simulink model "比例导引"  (R2023b)
settings: Solver=ode4  StartTime=0.0  StopTime=20  FixedStep=0.00005  RelTol=1e-3
settings Model: Creator=PC  LastModifiedBy=PC
settings DataIOCC: ReturnWorkspaceOutputs=off

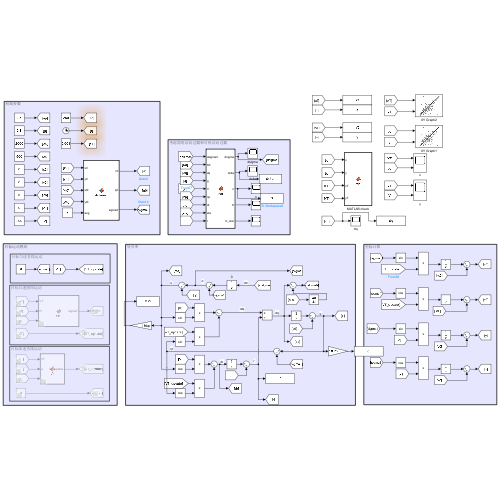
[thumbnail: Simulink's stored preview of the top-level diagram]
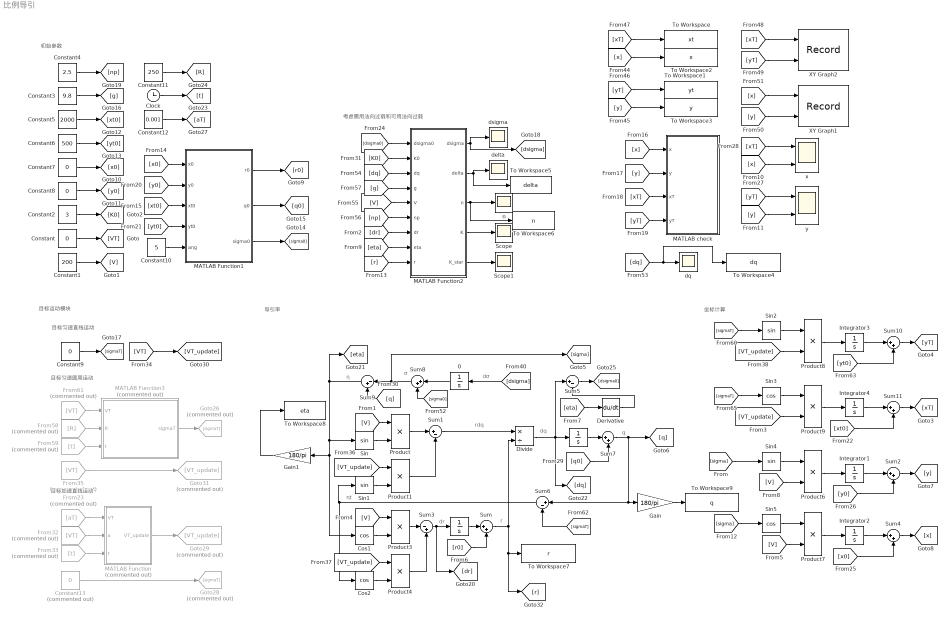
== system 比例导引 ==
  note: 目标加速直线运动
  note: 目标匀速圆周运动
  note: 目标匀速直线运动
  note: 目标运动模块
  note: 初始参数
  note: 导引率
  note: 坐标计算
  note: 考虑需用法向过载和可用法向过载
  note: rdq
  note: σ
  note: q
  note: dσ
  note: dq
  note: r
  note: dr
  note: η
  note: ηt
  " " : Integrator
  "  " : Integrator
  0 : Integrator
  Clock : Clock
  Constant{,7..9} (4 alike) : Constant  Value=0
  Constant1 : Constant  Value=200
  Constant10 : Constant  Value=5
  Constant11 : Constant  Value=250
  Constant12 : Constant  Value=0.001
  Constant13 : Constant  Commented=on  Value=0
  Constant2 : Constant  Value=3
  Constant3 : Constant  Value=9.8
  Constant4 : Constant  Value=2.5
  Constant5 : Constant  Value=2000
  Constant6 : Constant  Value=500
  Cos1 : Trigonometry  Operator=cos
  Cos2 : Trigonometry  Operator=cos
  Derivative : Derivative
  Divide : Product  Inputs=*/
  From23 : From  Commented=on  GotoTag=aT
  From32 : From  Commented=on  GotoTag=VT
  From33 : From  Commented=on  GotoTag=t
  From35 : From  Commented=on  GotoTag=VT
  From58 : From  Commented=on  GotoTag=R
  From59 : From  Commented=on  GotoTag=t
  From61 : From  Commented=on  GotoTag=VT
  Gain : Gain  Gain=180/pi
  Gain1 : Gain  Gain=180/pi
  Goto26 : Goto  Commented=on  GotoTag=sigmaT
  Goto28 : Goto  Commented=on  GotoTag=sigmaT
  Goto29 : Goto  Commented=on  GotoTag=VT_update
  Goto31 : Goto  Commented=on  GotoTag=VT_update
  Integrator{1..4} (4 alike) : Integrator
  MATLAB Function : MATLAB Function  Commented=on  TreatAsAtomicUnit=on
  MATLAB Function1 : MATLAB Function  TreatAsAtomicUnit=on
  MATLAB Function2 : MATLAB Function  TreatAsAtomicUnit=on
  MATLAB Function3 : MATLAB Function  Commented=on  TreatAsAtomicUnit=on
  MATLAB check : MATLAB Function  TreatAsAtomicUnit=on
  Product{,1,3..4,6..9} (8 alike) : Product
  Scope : Scope
  Scope1 : Scope
  Sin{,1..2,4} (4 alike) : Trigonometry
  Sin3 : Trigonometry  Operator=cos
  Sin5 : Trigonometry  Operator=cos
  Sum{,2,4,7..8,10..11} (7 alike) : Sum  Inputs=|++
  Sum1 : Sum  Inputs=|+-
  Sum3 : Sum  Inputs=|-+
  Sum5 : Sum  Inputs=|+-
  Sum6 : Sum  Inputs=|+-
  Sum9 : Sum  Inputs=|-+
  To Workspace : ToWorkspace  VariableName=xt  SaveFormat=Timeseries  SampleTime=-1
  To Workspace1 : ToWorkspace  VariableName=yt  SaveFormat=Timeseries  SampleTime=-1
  To Workspace2 : ToWorkspace  VariableName=x  SaveFormat=Timeseries  SampleTime=-1
  To Workspace3 : ToWorkspace  VariableName=y  SaveFormat=Timeseries  SampleTime=-1
  To Workspace4 : ToWorkspace  VariableName=dq  SaveFormat=Timeseries  SampleTime=-1
  To Workspace5 : ToWorkspace  VariableName=delta  SaveFormat=Timeseries  SampleTime=-1
  To Workspace6 : ToWorkspace  VariableName=n  SaveFormat=Timeseries  SampleTime=-1
  To Workspace7 : ToWorkspace  VariableName=r  SaveFormat=Timeseries  SampleTime=-1
  To Workspace8 : ToWorkspace  VariableName=eta  SaveFormat=Timeseries  SampleTime=-1
  To Workspace9 : ToWorkspace  VariableName=q  SaveFormat=Timeseries  SampleTime=-1
  XY Graph1 : Record  FileSettingsInternal="{\"entries\":[{\"content\":{\"excelSettings\":{\"content\":{},\"type\":\"Streamout.ExcelSettings\"}},\"type\":\"Streamout.FileSettingStorage\",\"uuid\":\"\"}],\"packageUris\":[\"http:\\/\\/schema.mathworks.com\\/mf0\\/streamout_blocks\\/R2020a\"],\"version\":\"1.0\"}"  Layout=[1 1]  SignalsInternal="{\"entries\":[{\"content\":{\"signals\":[{\"content\":{\"blockPath\":[],\"dimensions\":[1],\"domain\":\"\",\"lineColor\":\"#edb120\",\"plots\":[1],\"port\":1,\"sid\":[\"\"],\"signalID\":16369,\"signalName\":\"From51\"},\"type\":\"RecordBlkView.Signal\",\"uuid\":\"\"},{\"content\":{\"blockPath\":[],\"dimensions\":[1],\"domain\":\"\",\"lineColor\":\"#7e2f8e\",\"plots\":[1],\"port\":2,\"sid\":[\"\"],\"signalID\":16373,\"signalName\":\"From50\"},\"type\":\"RecordBlkView.Signal\",\"uuid\":\"\"}]},\"type\":\"RecordBlkView.InputSignals\",\"uuid\":\"\"}],\"packageUris\":[\"http:\\/\\/schema.mathworks.com\\/mf0\\/streamout_blocks\\/R2020a\"],\"version\":\"1.0\"}"  VisualizationBindings="{\"xyplotplugin\":{\"info\":[{\"series\":[{\"bindingParametersList\":[{\"parameter\":\"X-Axis\",\"signalID\":16369,\"signalName\":\"From51\"},{\"parameter\":\"Y-Axis\",\"signalID\":16373,\"signalName\":\"From50\"}],\"seriesID\":6684}],\"subplotID\":1}]}}"  CompatibilityTag=XY
  XY Graph2 : Record  FileSettingsInternal="{\"entries\":[{\"content\":{\"excelSettings\":{\"content\":{},\"type\":\"Streamout.ExcelSettings\"}},\"type\":\"Streamout.FileSettingStorage\",\"uuid\":\"\"}],\"packageUris\":[\"http:\\/\\/schema.mathworks.com\\/mf0\\/streamout_blocks\\/R2020a\"],\"version\":\"1.0\"}"  Layout=[1 1]  SignalsInternal="{\"entries\":[{\"content\":{\"signals\":[{\"content\":{\"blockPath\":[],\"dimensions\":[1],\"domain\":\"\",\"lineColor\":\"#edb120\",\"plots\":[1],\"port\":1,\"sid\":[\"\"],\"signalID\":16377,\"signalName\":\"From48\"},\"type\":\"RecordBlkView.Signal\",\"uuid\":\"\"},{\"content\":{\"blockPath\":[],\"dimensions\":[1],\"domain\":\"\",\"lineColor\":\"#7e2f8e\",\"plots\":[1],\"port\":2,\"sid\":[\"\"],\"signalID\":16381,\"signalName\":\"From49\"},\"type\":\"RecordBlkView.Signal\",\"uuid\":\"\"}]},\"type\":\"RecordBlkView.InputSignals\",\"uuid\":\"\"}],\"packageUris\":[\"http:\\/\\/schema.mathworks.com\\/mf0\\/streamout_blocks\\/R2020a\"],\"version\":\"1.0\"}"  VisualizationBindings="{\"xyplotplugin\":{\"info\":[{\"series\":[{\"bindingParametersList\":[{\"parameter\":\"X-Axis\",\"signalID\":16377,\"signalName\":\"From48\"},{\"parameter\":\"Y-Axis\",\"signalID\":16381,\"signalName\":\"From49\"}],\"seriesID\":60953}],\"subplotID\":1}]}}"  CompatibilityTag=XY
  delta : Scope
  dq : Scope
  dsigma : Scope
  n : Scope
  x : Scope  NumInputPorts=2
  y : Scope  NumInputPorts=2
  wires:
  Constant/1 -> [VT]
  Sin/1 -> Product/2
  [V] -> Product/1
  Sin1/1 -> Product1/2
  [VT_update] -> Product1/1
  [VT_update] -> Product4/1
  [V] -> Product3/1
  Cos1/1 -> Product3/2
  Cos2/1 -> Product4/2
  Product3/1 -> Sum3/1
  Product4/1 -> Sum3/2
  Sum3/1 -> [dr], " "/1
  Sum1/1 -> Divide/1
  Product/1 -> Sum1/1
  Product1/1 -> Sum1/2
  Divide/1 -> "  "/1, Sum5/1, [dq]
  Constant1/1 -> [V]
  Constant2/1 -> [K0]
  Sin4/1 -> Product6/1
  [V] -> Product6/2
  Product6/1 -> Integrator1/1
  Sum2/1 -> [y]
  Sin5/1 -> Product7/1
  [V] -> Product7/2
  Sum4/1 -> [x]
  Product7/1 -> Integrator2/1
  [x] -> MATLAB check/1(x)
  [y] -> MATLAB check/2(y)
  [xT] -> MATLAB check/3(xT)
  [yT] -> MATLAB check/4(yT)
  " "/1 -> Sum/1
  Sum/1 -> [r], To Workspace7/1, Divide/2
  [r0] -> Sum/2
  MATLAB Function1/1(r0) -> [r0]
  Constant7/1 -> [x0]
  Constant8/1 -> [y0]
  Constant5/1 -> [xt0]
  Constant6/1 -> [yt0]
  [y0] -> MATLAB Function1/2(y0)
  [x0] -> MATLAB Function1/1(x0)
  [xt0] -> MATLAB Function1/3(xt0)
  [yt0] -> MATLAB Function1/4(yt0)
  Integrator1/1 -> Sum2/1
  Integrator2/1 -> Sum4/1
  [sigma] -> Sin4/1
  [sigma] -> Sin5/1
  [y0] -> Sum2/2
  [x0] -> Sum4/2
  [yT] -> y/1
  [y] -> y/2
  "  "/1 -> Sum7/1
  Sum7/1 -> [q], Sum6/1, Gain/1
  [q0] -> Sum7/2
  0/1 -> Sum8/1
  Sum8/1 -> [sigma], Sum9/1
  [q] -> Sum9/2
  Sum9/1 -> Gain1/1, Cos1/1, Sin/1, [eta]
  [xT] -> x/1
  [x] -> x/2
  Constant3/1 -> [g]
  Constant4/1 -> [np]
  [xT] -> To Workspace/1
  [yT] -> To Workspace1/1
  [x] -> To Workspace2/1
  [y] -> To Workspace3/1
  [xT] -> XY Graph2/1
  [yT] -> XY Graph2/2
  [y] -> XY Graph1/2
  [x] -> XY Graph1/1
  MATLAB Function1/2(q0) -> [q0]
  [dq] -> To Workspace4/1, dq/1
  [sigma0] -> Sum8/2
  Constant10/1 -> MATLAB Function1/5(ang)
  MATLAB Function1/3(sigma0) -> [sigma0]
  [dsigma] -> 0/1
  [K0] -> MATLAB Function2/2(K0)
  [V] -> MATLAB Function2/5(V)
  [dq] -> MATLAB Function2/3(dq)
  [dsigma0] -> MATLAB Function2/1(dsigma0)
  [np] -> MATLAB Function2/6(np)
  [g] -> MATLAB Function2/4(g)
  Constant11/1 -> [R]
  Clock/1 -> [t]
  From58/1 -> MATLAB Function3/2(R)
  From59/1 -> MATLAB Function3/3(t)
  From61/1 -> MATLAB Function3/1(VT)
  [sigmaT] -> Sum6/2
  Sum6/1 -> Cos2/1, Sin1/1
  Constant9/1 -> [sigmaT]
  MATLAB Function3/1(sigmaT) -> Goto26/1
  Integrator3/1 -> Sum10/1
  Sum10/1 -> [yT]
  [VT_update] -> Product8/2
  Sin2/1 -> Product8/1
  [sigmaT] -> Sin2/1
  Product8/1 -> Integrator3/1
  [yt0] -> Sum10/2
  [xt0] -> Sum11/2
  Sin3/1 -> Product9/1
  [sigmaT] -> Sin3/1
  Product9/1 -> Integrator4/1
  Integrator4/1 -> Sum11/1
  [VT_update] -> Product9/2
  Sum11/1 -> [xT]
  [dr] -> MATLAB Function2/7(dr)
  [eta] -> MATLAB Function2/8(eta)
  MATLAB Function2/1(dsigma) -> [dsigma], dsigma/1
  Sum5/1 -> [dsigma0]
  [eta] -> Derivative/1
  Derivative/1 -> Sum5/2
  Constant12/1 -> [aT]
  From33/1 -> MATLAB Function/3(t)
  From32/1 -> MATLAB Function/2(a)
  From23/1 -> MATLAB Function/1(VT)
  Constant13/1 -> Goto28/1
  MATLAB Function/1(VT_update) -> Goto29/1
  [VT] -> [VT_update]
  From35/1 -> Goto31/1
  MATLAB Function2/2(delta) -> To Workspace5/1, delta/1
  MATLAB Function2/3(n) -> To Workspace6/1, n/1
  MATLAB Function2/4(K) -> Scope/1
  MATLAB Function2/5(K_star) -> Scope1/1
  [r] -> MATLAB Function2/9(r)
  Gain/1 -> To Workspace9/1
  Gain1/1 -> To Workspace8/1

== matlab function 比例导引/MATLAB check ==
  data: x input; y input; xT input; yT input
function  fcn(x,y,xT,yT)
if  (abs(x-xT)<0.1) && (abs(y-yT)<0.1) 
    error('hit!');
end

== matlab function 比例导引/MATLAB Function ==
  data: VT input; VT_update output; a input; t input
function VT_update = Vt(VT,a,t)
VT_update=VT+a*t;

== matlab function 比例导引/MATLAB Function1 ==
  data: x0 input; r0 output; y0 input; xt0 input; yt0 input; q0 output; ang input; sigma0 output
function [r0,q0,sigma0] = distance(x0,y0,xt0,yt0,ang)
r02=(xt0-x0)^2+(yt0-y0)^2;
r0=sqrt(r02);
q0=atan((yt0-y0)/(xt0-x0));
if (q0<=10*pi/180)
    sigma0=ang*pi/180+q0;
else
    sigma0=q0;
end

== matlab function 比例导引/MATLAB Function2 ==
  data: dsigma0 input; K0 input; dq input; g input; V input; np input; dr input; eta input; dsigma output; delta output; n output; K output; K_star output; r input
function [dsigma,delta,n,K,K_star]  = fcn(dsigma0,K0,dq,g,V,np,dr,eta,r)
n=V*dsigma0/g;
if abs(n)>=np
    if n>=0
        dsigma=np*g/V;
        K=abs(dsigma/dq);
        n=np;
    else
        dsigma=-np*g/V;
        K=abs(dsigma/dq);
        n=-np;
    end
else
    dsigma=K0*dq;
    K=K0;
end

% 
% if r<=50
%     dsigma=0;
% end
% K=K0;
K_star=2*abs(dr)/(V*cos(eta));

% K=K_star;
% dsigma=K*dq;

delta=K_star-K;
% dsigma=K*dq;
% dsigma=K_star*dq;
% if abs(K)<=K_star
%     K=K_star;
% end

== matlab function 比例导引/MATLAB Function3 ==
  data: VT input; sigmaT output; R input; t input
function sigmaT  = fcn(VT,R,t)
wT=VT/R;
sigmaT=wT*t;
